simulink model "scenario1_more_complex_new"  (R2020b)
settings: Solver=FixedStepAuto  StartTime=0.0  StopTime=60.0  FixedStep=1e-2  RelTol=1e-3
libraries: simulink x3
settings Model: Creator=Admin  LastModifiedBy=Admin

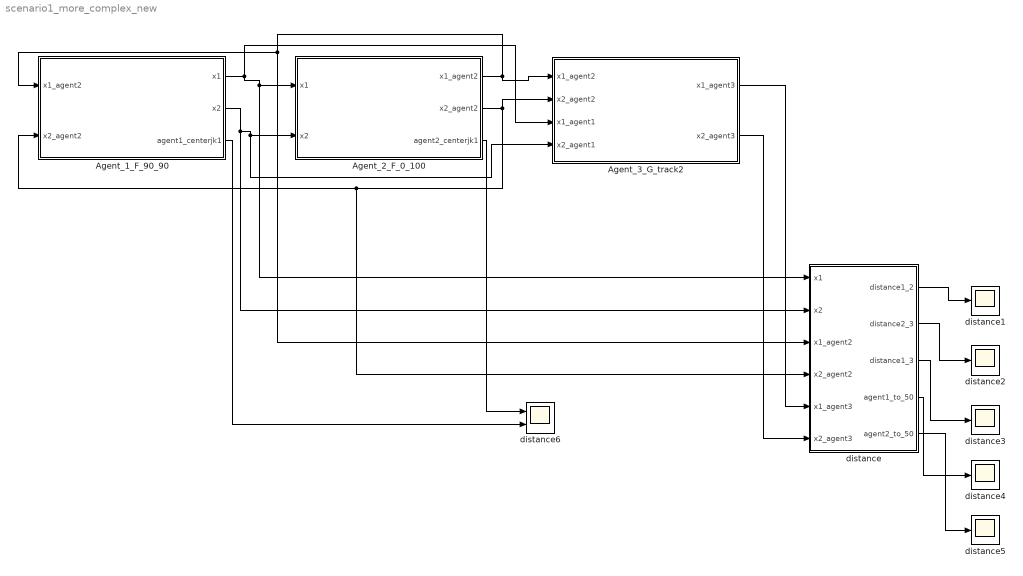
== system scenario1_more_complex_new ==
  Agent_1_F_90_90 : Subsystem
  Agent_2_F_0_100 : Subsystem
  Agent_3_G_track2 : Subsystem
  "distance " : MATLAB Function  TreatAsAtomicUnit=on
  distance{1..5} (5 alike) : Scope
  distance6 : Scope  NumInputPorts=2
  wires:
  Agent_1_F_90_90/1(x1) -> "distance "/1(x1), Agent_2_F_0_100/1(x1), Agent_3_G_track2/3(x1_agent1)
  Agent_1_F_90_90/2(x2) -> "distance "/2(x2), Agent_3_G_track2/4(x2_agent1), Agent_2_F_0_100/2(x2)
  Agent_2_F_0_100/1(x1_agent2) -> Agent_3_G_track2/1(x1_agent2), "distance "/3(x1_agent2), Agent_1_F_90_90/1(x1_agent2)
  Agent_2_F_0_100/2(x2_agent2) -> "distance "/4(x2_agent2), Agent_1_F_90_90/2(x2_agent2), Agent_3_G_track2/2(x2_agent2)
  "distance "/1(distance1_2) -> distance1/1
  Agent_3_G_track2/1(x1_agent3) -> "distance "/5(x1_agent3)
  Agent_3_G_track2/2(x2_agent3) -> "distance "/6(x2_agent3)
  "distance "/2(distance2_3) -> distance2/1
  "distance "/3(distance1_3) -> distance3/1
  "distance "/4(agent1_to_50) -> distance4/1
  "distance "/5(agent2_to_50) -> distance5/1
  Agent_2_F_0_100/3(agent2_centerjk1) -> distance6/1
  Agent_1_F_90_90/3(agent1_centerjk1) -> distance6/2

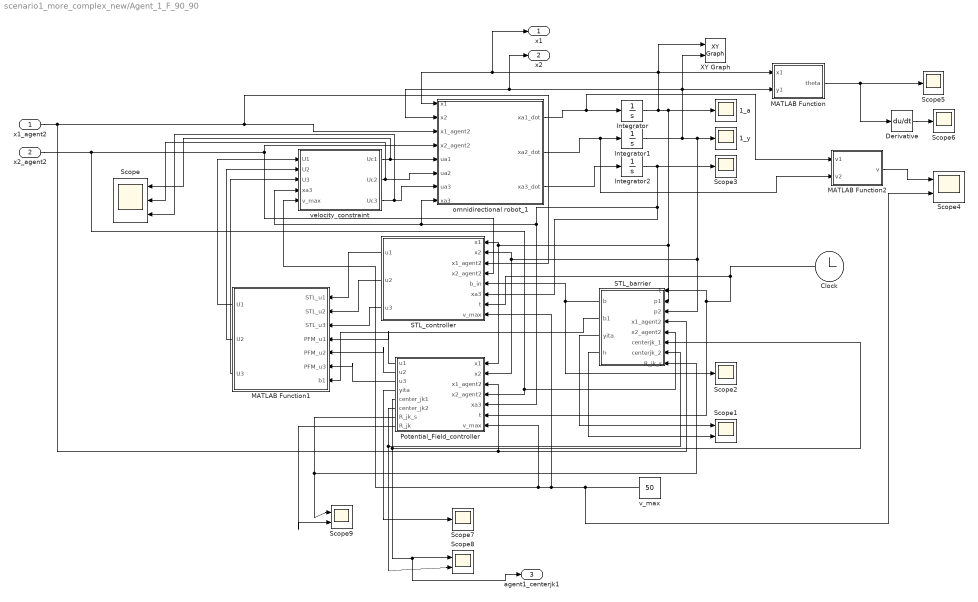
== system scenario1_more_complex_new/Agent_1_F_90_90 ==
  x1_agent2 : Inport
  x2_agent2 : Inport  Port=2
  1_a : Scope
  1_y : Scope
  Clock : Clock
  Derivative : Derivative
  Integrator : Integrator
  Integrator1 : Integrator
  Integrator2 : Integrator
  MATLAB Function : MATLAB Function  TreatAsAtomicUnit=on
  MATLAB Function1 : MATLAB Function  TreatAsAtomicUnit=on
  MATLAB Function2 : MATLAB Function  TreatAsAtomicUnit=on
  Potential_Field_controller : MATLAB Function  TreatAsAtomicUnit=on
  "STL_barrier " : MATLAB Function  TreatAsAtomicUnit=on
  STL_controller : MATLAB Function  TreatAsAtomicUnit=on
  Scope : Scope  NumInputPorts=3
  Scope{1,4,8..9} (4 alike) : Scope  NumInputPorts=2
  Scope{2..3,5..7} (5 alike) : Scope
  XY Graph : simulink/Sinks/XY Graph  xmin=-15  xmax=100  ymin=-15  ymax=100  st=0.01
  omnidirectional robot_1 : MATLAB Function  TreatAsAtomicUnit=on
  v_max : Constant  Value=50
  velocity_constraint : MATLAB Function  TreatAsAtomicUnit=on
  x1 : Outport
  x2 : Outport  Port=2
  agent1_centerjk1 : Outport  Port=3
  wires:
  MATLAB Function/1(theta) -> Derivative/1, Scope5/1
  MATLAB Function1/3(U3) -> velocity_constraint/3(U3)
  "STL_barrier "/1(b) -> Scope2/1, STL_controller/5(b_in)
  Potential_Field_controller/3(u3) -> MATLAB Function1/6(PFM_u3)
  STL_controller/2(u2) -> MATLAB Function1/2(STL_u2)
  Integrator2/1 -> Potential_Field_controller/5(xa3), velocity_constraint/4(xa3), omnidirectional robot_1/8(xa3), STL_controller/6(xa3), Scope3/1
  Integrator1/1 -> x2/1, omnidirectional robot_1/2(x2), MATLAB Function/2(y1), XY Graph/2, "STL_barrier "/3(p2), Potential_Field_controller/2(x2), STL_controller/2(x2), 1_y/1
  Potential_Field_controller/1(u1) -> MATLAB Function1/4(PFM_u1)
  "STL_barrier "/3(yita) -> Scope1/1
  "STL_barrier "/4(h) -> Scope1/2
  omnidirectional robot_1/1(xa1_dot) -> MATLAB Function2/1(v1), Integrator/1
  STL_controller/1(u1) -> MATLAB Function1/1(STL_u1)
  "STL_barrier "/2(b1) -> MATLAB Function1/7(b1)
  STL_controller/3(u3) -> MATLAB Function1/3(STL_u3)
  omnidirectional robot_1/3(xa3_dot) -> Integrator2/1
  Clock/1 -> Potential_Field_controller/6(t), "STL_barrier "/1(t), STL_controller/7(t)
  MATLAB Function1/1(U1) -> velocity_constraint/1(U1)
  Derivative/1 -> Scope6/1
  omnidirectional robot_1/2(xa2_dot) -> MATLAB Function2/2(v2), Integrator1/1
  Potential_Field_controller/2(u2) -> MATLAB Function1/5(PFM_u2)
  MATLAB Function1/2(U2) -> velocity_constraint/2(U2)
  Integrator/1 -> x1/1, omnidirectional robot_1/1(x1), MATLAB Function/1(x1), XY Graph/1, "STL_barrier "/2(p1), Potential_Field_controller/1(x1), STL_controller/1(x1), 1_a/1
  x1_agent2/1 -> "STL_barrier "/4(x1_agent2), Potential_Field_controller/3(x1_agent2), STL_controller/3(x1_agent2), omnidirectional robot_1/3(x1_agent2)
  x2_agent2/1 -> Potential_Field_controller/4(x2_agent2), "STL_barrier "/5(x2_agent2), omnidirectional robot_1/4(x2_agent2), STL_controller/4(x2_agent2)
  MATLAB Function2/1(v) -> Scope4/1
  velocity_constraint/1(Uc1) -> Scope/1, omnidirectional robot_1/5(ua1)
  velocity_constraint/2(Uc2) -> omnidirectional robot_1/6(ua2), Scope/2
  velocity_constraint/3(Uc3) -> Scope/3, omnidirectional robot_1/7(ua3)
  v_max/1 -> Scope4/2, STL_controller/8(v_max), velocity_constraint/5(v_max), Potential_Field_controller/7(v_max)
  Potential_Field_controller/4(yita) -> Scope7/1
  Potential_Field_controller/6(center_jk2) -> "STL_barrier "/7(centerjk_2), Scope8/2
  Potential_Field_controller/7(R_jk_s) -> "STL_barrier "/8(R_jk_s), Scope9/1
  Potential_Field_controller/8(R_jk) -> Scope9/2
  Potential_Field_controller/5(center_jk1) -> agent1_centerjk1/1, Scope8/1, "STL_barrier "/6(centerjk_1)

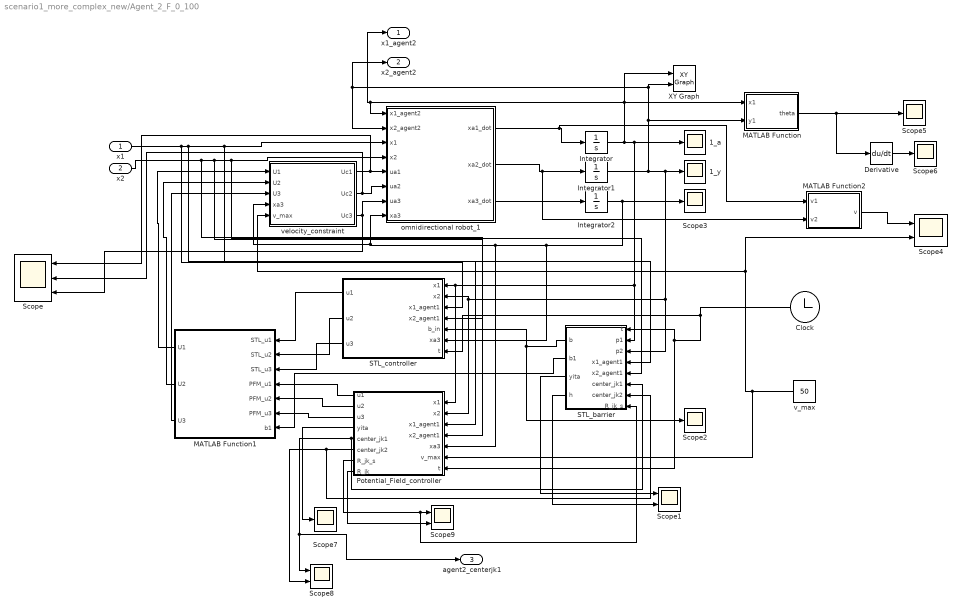
== system scenario1_more_complex_new/Agent_2_F_0_100 ==
  x1 : Inport
  x2 : Inport  Port=2
  1_a : Scope
  1_y : Scope
  Clock : Clock
  Derivative : Derivative
  Integrator : Integrator  InitialCondition=100
  Integrator1 : Integrator
  Integrator2 : Integrator
  MATLAB Function : MATLAB Function  TreatAsAtomicUnit=on
  MATLAB Function1 : MATLAB Function  TreatAsAtomicUnit=on
  MATLAB Function2 : MATLAB Function  TreatAsAtomicUnit=on
  Potential_Field_controller : MATLAB Function  TreatAsAtomicUnit=on
  "STL_barrier " : MATLAB Function  TreatAsAtomicUnit=on
  STL_controller : MATLAB Function  TreatAsAtomicUnit=on
  Scope : Scope  NumInputPorts=3
  Scope{1,4,8..9} (4 alike) : Scope  NumInputPorts=2
  Scope{2..3,5..7} (5 alike) : Scope
  XY Graph : simulink/Sinks/XY Graph  xmin=-15  xmax=100  ymin=-15  ymax=100  st=0.01
  omnidirectional robot_1 : MATLAB Function  TreatAsAtomicUnit=on
  v_max : Constant  Value=50
  velocity_constraint : MATLAB Function  TreatAsAtomicUnit=on
  x1_agent2 : Outport
  x2_agent2 : Outport  Port=2
  agent2_centerjk1 : Outport  Port=3
  wires:
  MATLAB Function/1(theta) -> Derivative/1, Scope5/1
  MATLAB Function1/3(U3) -> velocity_constraint/3(U3)
  "STL_barrier "/1(b) -> Scope2/1, STL_controller/5(b_in)
  Potential_Field_controller/3(u3) -> MATLAB Function1/6(PFM_u3)
  STL_controller/2(u2) -> MATLAB Function1/2(STL_u2)
  Integrator2/1 -> Potential_Field_controller/5(xa3), velocity_constraint/4(xa3), omnidirectional robot_1/8(xa3), STL_controller/6(xa3), Scope3/1
  Integrator1/1 -> x2_agent2/1, omnidirectional robot_1/2(x2_agent2), XY Graph/2, MATLAB Function/2(y1), "STL_barrier "/3(p2), Potential_Field_controller/2(x2), STL_controller/2(x2), 1_y/1
  Potential_Field_controller/1(u1) -> MATLAB Function1/4(PFM_u1)
  Integrator/1 -> x1_agent2/1, omnidirectional robot_1/1(x1_agent2), MATLAB Function/1(x1), XY Graph/1, "STL_barrier "/2(p1), Potential_Field_controller/1(x1), STL_controller/1(x1), 1_a/1
  "STL_barrier "/3(yita) -> Scope1/1
  "STL_barrier "/4(h) -> Scope1/2
  omnidirectional robot_1/1(xa1_dot) -> MATLAB Function2/1(v1), Integrator/1
  STL_controller/1(u1) -> MATLAB Function1/1(STL_u1)
  "STL_barrier "/2(b1) -> MATLAB Function1/7(b1)
  STL_controller/3(u3) -> MATLAB Function1/3(STL_u3)
  omnidirectional robot_1/3(xa3_dot) -> Integrator2/1
  Clock/1 -> Potential_Field_controller/7(t), "STL_barrier "/1(t), STL_controller/7(t)
  MATLAB Function1/1(U1) -> velocity_constraint/1(U1)
  Derivative/1 -> Scope6/1
  omnidirectional robot_1/2(xa2_dot) -> MATLAB Function2/2(v2), Integrator1/1
  Potential_Field_controller/2(u2) -> MATLAB Function1/5(PFM_u2)
  MATLAB Function1/2(U2) -> velocity_constraint/2(U2)
  x1/1 -> STL_controller/3(x1_agent1), Potential_Field_controller/3(x1_agent1), "STL_barrier "/4(x1_agent1), omnidirectional robot_1/3(x1)
  x2/1 -> STL_controller/4(x2_agent1), Potential_Field_controller/4(x2_agent1), "STL_barrier "/5(x2_agent1), omnidirectional robot_1/4(x2)
  MATLAB Function2/1(v) -> Scope4/1
  v_max/1 -> Potential_Field_controller/6(v_max), Scope4/2, velocity_constraint/5(v_max)
  velocity_constraint/1(Uc1) -> Scope/1, omnidirectional robot_1/5(ua1)
  velocity_constraint/2(Uc2) -> Scope/2, omnidirectional robot_1/6(ua2)
  velocity_constraint/3(Uc3) -> Scope/3, omnidirectional robot_1/7(ua3)
  Potential_Field_controller/4(yita) -> Scope7/1
  Potential_Field_controller/5(center_jk1) -> "STL_barrier "/6(center_jk1), Scope8/1, agent2_centerjk1/1
  Potential_Field_controller/6(center_jk2) -> "STL_barrier "/7(center_jk2), Scope8/2
  Potential_Field_controller/7(R_jk_s) -> "STL_barrier "/8(R_jk_s), Scope9/1
  Potential_Field_controller/8(R_jk) -> Scope9/2

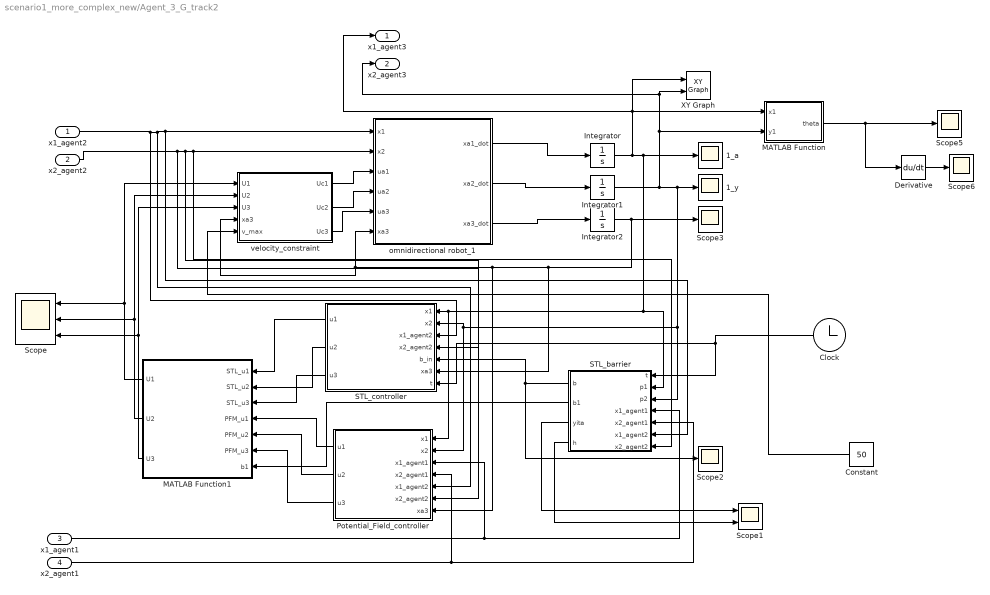
== system scenario1_more_complex_new/Agent_3_G_track2 ==
  x1_agent2 : Inport
  x2_agent2 : Inport  Port=2
  x1_agent1 : Inport  Port=3
  x2_agent1 : Inport  Port=4
  1_a : Scope
  1_y : Scope
  Clock : Clock
  Constant : Constant  Value=50
  Derivative : Derivative
  Integrator : Integrator  InitialCondition=100
  Integrator1 : Integrator  InitialCondition=50
  Integrator2 : Integrator
  MATLAB Function : MATLAB Function  TreatAsAtomicUnit=on
  MATLAB Function1 : MATLAB Function  TreatAsAtomicUnit=on
  Potential_Field_controller : MATLAB Function  TreatAsAtomicUnit=on
  "STL_barrier " : MATLAB Function  TreatAsAtomicUnit=on
  STL_controller : MATLAB Function  TreatAsAtomicUnit=on
  Scope : Scope  NumInputPorts=3
  Scope1 : Scope  NumInputPorts=2
  Scope{2..3,5..6} (4 alike) : Scope
  XY Graph : simulink/Sinks/XY Graph  xmin=-15  xmax=100  ymin=-15  ymax=100  st=0.01
  omnidirectional robot_1 : MATLAB Function  TreatAsAtomicUnit=on
  velocity_constraint : MATLAB Function  TreatAsAtomicUnit=on
  x1_agent3 : Outport
  x2_agent3 : Outport  Port=2
  wires:
  MATLAB Function/1(theta) -> Derivative/1, Scope5/1
  MATLAB Function1/3(U3) -> velocity_constraint/3(U3), Scope/3
  "STL_barrier "/1(b) -> STL_controller/5(b_in), Scope2/1
  Potential_Field_controller/3(u3) -> MATLAB Function1/6(PFM_u3)
  STL_controller/2(u2) -> MATLAB Function1/2(STL_u2)
  Integrator2/1 -> Potential_Field_controller/7(xa3), omnidirectional robot_1/6(xa3), velocity_constraint/4(xa3), STL_controller/6(xa3), Scope3/1
  Integrator1/1 -> x2_agent3/1, XY Graph/2, MATLAB Function/2(y1), "STL_barrier "/3(p2), Potential_Field_controller/2(x2), STL_controller/2(x2), 1_y/1
  Potential_Field_controller/1(u1) -> MATLAB Function1/4(PFM_u1)
  Integrator/1 -> x1_agent3/1, MATLAB Function/1(x1), XY Graph/1, "STL_barrier "/2(p1), Potential_Field_controller/1(x1), STL_controller/1(x1), 1_a/1
  "STL_barrier "/3(yita) -> Scope1/1
  "STL_barrier "/4(h) -> Scope1/2
  omnidirectional robot_1/1(xa1_dot) -> Integrator/1
  STL_controller/1(u1) -> MATLAB Function1/1(STL_u1)
  "STL_barrier "/2(b1) -> MATLAB Function1/7(b1)
  STL_controller/3(u3) -> MATLAB Function1/3(STL_u3)
  omnidirectional robot_1/3(xa3_dot) -> Integrator2/1
  Clock/1 -> "STL_barrier "/1(t), STL_controller/7(t)
  MATLAB Function1/1(U1) -> velocity_constraint/1(U1), Scope/1
  Derivative/1 -> Scope6/1
  omnidirectional robot_1/2(xa2_dot) -> Integrator1/1
  Potential_Field_controller/2(u2) -> MATLAB Function1/5(PFM_u2)
  MATLAB Function1/2(U2) -> velocity_constraint/2(U2), Scope/2
  x1_agent2/1 -> STL_controller/3(x1_agent2), Potential_Field_controller/5(x1_agent2), "STL_barrier "/6(x1_agent2), omnidirectional robot_1/1(x1)
  x2_agent2/1 -> STL_controller/4(x2_agent2), Potential_Field_controller/6(x2_agent2), "STL_barrier "/7(x2_agent2), omnidirectional robot_1/2(x2)
  x1_agent1/1 -> Potential_Field_controller/3(x1_agent1), "STL_barrier "/4(x1_agent1)
  x2_agent1/1 -> Potential_Field_controller/4(x2_agent1), "STL_barrier "/5(x2_agent1)
  Constant/1 -> velocity_constraint/5(v_max)
  velocity_constraint/1(Uc1) -> omnidirectional robot_1/3(ua1)
  velocity_constraint/2(Uc2) -> omnidirectional robot_1/4(ua2)
  velocity_constraint/3(Uc3) -> omnidirectional robot_1/5(ua3)

== matlab function scenario1_more_complex_new/Agent_2_F_0_100/MATLAB Function ==
  data: x1 input; theta output; y1 input
function theta = fcn(x1, y1)
theta=atan2(y1,x1);

== matlab function scenario1_more_complex_new/Agent_2_F_0_100/MATLAB Function1 ==
  data: STL_u1 input; U1 output; STL_u2 input; STL_u3 input; PFM_u1 input; PFM_u2 input; PFM_u3 input; b1 input; U2 output; U3 output
function [U1,U2,U3] = fcn(STL_u1,STL_u2,STL_u3,PFM_u1,PFM_u2,PFM_u3,b1)
U_goal=[STL_u1;STL_u2;STL_u3];
U_obs=[PFM_u1;PFM_u2;PFM_u3];
k=0.15;
lambda=1-exp(-k*max(b1,0));
U=lambda*U_goal+(1-lambda)*U_obs;
U1=0;U2=0;U3=0;
U1=U(1,1);
U2=U(2,1);
U3=U(3,1);

== matlab function scenario1_more_complex_new/distance  ==
  data: x1 input; distance1_2 output; x2 input; x1_agent2 input; x2_agent2 input; x1_agent3 input; x2_agent3 input; distance2_3 output; distance1_3 output; agent1_to_50 output; agent2_to_50 output
function [distance1_2,distance2_3,distance1_3,agent1_to_50,agent2_to_50] = fcn(x1,x2,x1_agent2,x2_agent2,x1_agent3,x2_agent3)
distance1_2=sqrt((x1-x1_agent2)^2+(x2-x2_agent2)^2);
distance2_3=sqrt((x1_agent2-x1_agent3)^2+(x2_agent2-x2_agent3)^2);
distance1_3=sqrt((x1-x1_agent3)^2+(x2-x2_agent3)^2);
agent1_to_50=sqrt((x1-50)^2+(x2-50)^2);
agent2_to_50=sqrt((x1_agent2-50)^2+(x2_agent2-50)^2);

== matlab function scenario1_more_complex_new/Agent_2_F_0_100/STL_barrier  ==
  data: b output; b1 output; yita output; h output; t input; p1 input; p2 input; x1_agent1 input; x2_agent1 input; center_jk1 input; center_jk2 input; R_jk_s input
function [b,b1,yita,h] = fcn(t,p1,p2,x1_agent1, x2_agent1, center_jk1,center_jk2,R_jk_s)
if t<20
    d1=0;
    d2=100;
elseif t>=20 && t<40
    d1=90;
    d2=90;
else
    d1=0;
    d2=0;
end
    

obs1=50;
obs2=50;

if t<20
    b=145*exp(-0.24*t)+5-sqrt( (p1-d1)^2 + (p2-d2)^2 );
    yita=-145*exp(-0.24*t)+5;
    h=10-sqrt( (p1-d1)^2 + (p2-d2)^2 );
elseif t>=20 && t<40
   b=90*exp(-0.208*(t-20))+5-sqrt( (p1-d1)^2 + (p2-d2)^2 );
   yita=-90*exp(-0.208*(t-20))+5;
   h=10-sqrt( (p1-d1)^2 + (p2-d2)^2 );
else
   b=135*exp(-0.235*(t-40))+5-sqrt( (p1-d1)^2 + (p2-d2)^2 );
   yita=-135*exp(-0.235*(t-40))+5;
   h=10-sqrt( (p1-d1)^2 + (p2-d2)^2 );    
end
b11=sqrt( (p1-obs1)^2 + (p2-obs2)^2 )-20;%collision avoidence with (50,50)
b12=sqrt( (p1-x1_agent1)^2 + (p2-x2_agent1)^2 )-6;%collision avoidence with agent1
b13=sqrt( (p1-center_jk1)^2 + (p2-center_jk2)^2 )-R_jk_s;%collision avoidence with agent1
b14=sqrt( (p1-60)^2 + (p2-80)^2 )-15;
b15=sqrt( (p1-10)^2 + (p2-70)^2 )-10;
if R_jk_s==0
b1=-(1/20)*log(exp(-20*b11)+exp(-20*b12)+exp(-20*b14)+exp(-20*b15));%+log(2);
else
b1=-(1/20)*log(exp(-20*b11)+exp(-20*b12)+exp(-20*b13)+exp(-20*b14)+exp(-20*b15));%+log(2);
end

== matlab function scenario1_more_complex_new/Agent_2_F_0_100/STL_controller ==
  data: x1 input; x2 input; x1_agent1 input; x2_agent1 input; b_in input; u1 output; xa3 input; u2 output; u3 output; t input
function [u1,u2,u3]= fcn(x1, x2,x1_agent1,x2_agent1, b_in, xa3,t)
%Note：x are the position of agent2(myself), and x_agent1 is from another agent
coder.extrinsic('quadoptimizer');
%coder.extrinsic('save');
if t<20
d1=0; d2=100;
elseif t>=20 && t<40
d1=90; d2=90;
else
d1=0; d2=0;
end
partial_b=(1/2)*((x1-d1)^2+(x2-d2)^2)^(-1/2);
partial_b_x=[-2*partial_b*(x1-d1),-2*partial_b*(x2-d2),0];


Li=0.2;
Bi=[0,cos(pi/6),-cos(pi/6);
    -1,sin(pi/6),sin(pi/6);
    Li,Li,Li;];

R1=[cos(xa3),-sin(xa3),0;
    sin(xa3),cos(xa3),0;
    0,0,1;];
R=0.02;
gx=R1*inv(Bi')*R;

A=partial_b_x*gx;
% A=[A;-gx];

H=[1,0,0;0,1,0;0,0,1];
%H=[1];
if t<20
   b=2*b_in-0.24*125*exp(-0.24*t)-4;
elseif t>=20 && t<40
   b=2*b_in-0.208*90*exp(-0.208*(t-20))-4;
else
   b=2*b_in-0.235*135*exp(-0.235*(t-40))-4; 
end
% b=[b;5000;5000;5000];


u1=0;u2=0;u3=0;
U=quadoptimizer(H,b,A);

%U=quadprod(H,[],-A,b);

u1=U(1,1);
u2=U(2,1);
u3=U(3,1);

== matlab function scenario1_more_complex_new/Agent_2_F_0_100/omnidirectional robot_1 ==
  data: x1_agent2 input; x2_agent2 input; x1 input; x2 input; ua1 input; xa1_dot output; ua2 input; ua3 input; xa3 input; xa2_dot output; xa3_dot output
function [xa1_dot,xa2_dot,xa3_dot]= fcn(x1_agent2,x2_agent2,x1,x2,ua1,ua2,ua3,xa3)

Li=0.2;
Bi=[0,cos(pi/6),-cos(pi/6);
    -1,sin(pi/6),sin(pi/6);
    Li,Li,Li;];

R1=[cos(xa3),-sin(xa3),0;
    sin(xa3),cos(xa3),0;
    0,0,1;];
R=0.02;
A=R1*inv(Bi')*R*[ua1;ua2;ua3];
xa1_dot=A(1,1);
xa2_dot=A(2,1);
xa3_dot=A(3,1);

== matlab function scenario1_more_complex_new/Agent_2_F_0_100/Potential_Field_controller ==
  data: x1 input; x2 input; x1_agent1 input; x2_agent1 input; u1 output; xa3 input; u2 output; u3 output; v_max input; yita output; center_jk1 output; center_jk2 output; R_jk_s output; R_jk output; t input
function [u1,u2,u3,yita,center_jk1,center_jk2,R_jk_s,R_jk] = fcn(x1, x2, x1_agent1,x2_agent1, xa3,v_max,t)
coder.extrinsic('Calculate_gradient');
coder.extrinsic('Calculate_gradient_V2');
coder.extrinsic('Calculate_gradient_V1_yita');
coder.extrinsic('Calculate_gradient_static_d_1');
coder.extrinsic('Calculate_gradient_static_d_2');
coder.extrinsic('compute_convex_hull');
coder.extrinsic('PVF_optimizer');
coder.extrinsic('add_random');
yita=0;
center_jk1=0;center_jk2=0;
A1=[-1,0;0,-1];
if t<20
    F=[0,200];
elseif t>=20 && t<40
    F=[180,180];
else 
   F=[0,0]; 
end
obs=[50,50];
Robs_s=20;R1_s=6;
r_obs=16;d1=3;
R_jk_s=0;R_jk=0
distance=sqrt((x1-0)^2+(x2-100)^2);
gradient_x=0;gradient_y=0;
Dgradient_x=0;Dgradient_y=0;D1gradient_x=0;D1gradient_y=0;D2gradient_x=0;D2gradient_y=0;
[gradient_x,gradient_y]=Calculate_gradient(x1,x2,A1,F,50,50,Robs_s);
[Dgradient_x,Dgradient_y]=Calculate_gradient_V2(x1,x2,A1,F,x1_agent1,x2_agent1,R1_s);
[D1gradient_x,D1gradient_y]=Calculate_gradient_static_d_1(x1,x2,A1,F,60,85,15);
[D2gradient_x,D2gradient_y]=Calculate_gradient_static_d_2(x1,x2,A1,F,10,70,10);
agent_distance=sqrt((x1-x1_agent1)^2+(x2-x2_agent1)^2);%the distance between 1 and 2.
if t>20
gradient_x=gradient_x+D1gradient_x;
gradient_y=gradient_y+D1gradient_y;
else
gradient_x=gradient_x+D2gradient_x;
gradient_y=gradient_y+D2gradient_y;
end
% gradient_x=Gradient(1,1);
% gradient_y=Gradient(1,2);
gradient_z=0;

if agent_distance>50
     Gradient_all=[gradient_x;gradient_y;gradient_z];
else 
     gradient_x=gradient_x+Dgradient_x;
     gradient_y=gradient_y+Dgradient_y;
     Gradient_all=[gradient_x;gradient_y;gradient_z];
end
% if agent_distance>40
%     Gradient_all=[gradient_x;gradient_y;gradient_z];
% else %collision avoidence with agent 2
%      if sqrt((x1_agent1-obs(1,1))^2+(x2_agent1-obs(1,2))^2)>Robs_s+R1_s %compute if intersection happens,No intersecdtion
%          gradient_x=gradient_x+Dgradient_x;
%          gradient_y=gradient_y+Dgradient_y;
%          Gradient_all=[gradient_x;gradient_y;gradient_z];
%      else %intersecdtion happens
%          center_jk1=0; center_jk2=0; R_jk=0;flg_jk=0;
%          [center_jk1, center_jk2, R_jk,flg_jk]=compute_convex_hull(x1,x2,obs(1,1), obs(1,2), x1_agent1, x2_agent1,r_obs,d1);
%           if sqrt((x1-center_jk1)^2+(x2-center_jk2)^2)<R_jk %inside the convexhull
%                [Dgradient_x,Dgradient_y]=Calculate_gradient_V1(x1,x2,A1,F,x1_agent2,x2_agent2,R2_s*exp(-2*v_max*(t-t0)));
%                   gradient_x=gradient_x;%+Dgradient_x;
%                   gradient_y=gradient_y;%+Dgradient_y;
%                   Gradient_all=[gradient_x;gradient_y;gradient_z];
%                   center_jk1=10; center_jk2=0;
%           else %outside the convexhull
%               if flg_jk==1 %outside and nomial need to be built
%                R_jk_s=(R_jk/d1)*R1_s;  
%                    R_jk_s=sqrt((x1-center_jk1)^2+(x2-center_jk2)^2);
%                    R_jk_s=50;
%                    yita= ( (v_max+50*0.6+2)*R_jk^3 )/( 50*(1- (R_jk/R_jk_s) ) );
%                    Djkgradient_x=0;Djkgradient_y=0;
%                    [Djkgradient_x,Djkgradient_y]=Calculate_gradient_V1_yita(x1,x2,A1,F,center_jk1,center_jk2,R_jk_s,yita);
%                     gradient_x=gradient_x+Dgradient_x+Djkgradient_x;
%                     gradient_y=gradient_y+Dgradient_y+Djkgradient_y;
%                     Gradient_all=[gradient_x;gradient_y;gradient_z];
%               else %%outside and nomialdo not need to be built
%                     gradient_x=gradient_x+Dgradient_x;
%                     gradient_y=gradient_y+Dgradient_y;
%                     Gradient_all=[gradient_x;gradient_y;gradient_z];
%               end
%           end
%      end
% end
             

Li=0.2;
Bi=[0,cos(pi/6),-cos(pi/6);
    -1,sin(pi/6),sin(pi/6);
    Li,Li,Li;];

R1=[cos(xa3),-sin(xa3),0;
    sin(xa3),cos(xa3),0;
    0,0,1;];
R=0.02;

gx=R1*inv(Bi')*R;
A=Gradient_all'*gx;
% A=[A;-gx];

%H=[1];
%H=[1,0;0,1];
%H=[0,0,0;0,0,0;0,0,0];
% H=[1,0,0;0,1,0;0,0,1];
 H=(1/2)*gx'*gx;
b=[0];
% b=[0;5000;5000;5000];
Gain=50;
Gradient_final=Gain*Gradient_all;
F=[-2*gx'*Gradient_final];
%=[];
u1=0;u2=0;u3=0;
U=PVF_optimizer(H,b,A,F,distance,gradient_x,gradient_y);

u1=U(1,1);
u2=U(2,1);
u3=U(3,1);

== matlab function scenario1_more_complex_new/Agent_1_F_90_90/STL_barrier  ==
  data: b output; b1 output; yita output; h output; t input; p1 input; p2 input; x1_agent2 input; x2_agent2 input; centerjk_1 input; centerjk_2 input; R_jk_s input
function [b,b1,yita,h] = fcn(t,p1,p2, x1_agent2, x2_agent2,centerjk_1,centerjk_2,R_jk_s)
if t<20
    d1=90;
    d2=90;
elseif t>=20 && t<40
    d1=0;
    d2=100;
else
    d1=100;
    d2=0;  
end

obs1=50;
obs2=50;
if t<20
b=125*exp(-0.2295*t)+5-sqrt( (p1-d1)^2 + (p2-d2)^2 );
yita=-125*exp(-0.2295*t)+5;
h=10-sqrt( (p1-d1)^2 + (p2-d2)^2 );
elseif t>=20 && t<40
    b=90*exp(-0.208*(t-20))+5-sqrt( (p1-d1)^2 + (p2-d2)^2 );
   yita=-90*exp(-0.2295*(t-20))+5;
    h=10-sqrt( (p1-d1)^2 + (p2-d2)^2 );
else
   b=145*exp(-0.24*(t-40))+5-sqrt( (p1-d1)^2 + (p2-d2)^2 );
   yita=-145*exp(-0.24*(t-40))+5;
   h=10-sqrt( (p1-d1)^2 + (p2-d2)^2 );
end
b11=sqrt( (p1-x1_agent2)^2 + (p2-x2_agent2)^2 )-10 %collision avoidence with agent2
b12=sqrt( (p1-obs1)^2 + (p2-obs2)^2 )-20;%collision avoidence with obstacle (50,50)
b13=sqrt( (p1-centerjk_1)^2 + (p2-centerjk_2)^2 )-R_jk_s;%collision avoidence with nominal
b14=sqrt( (p1-60)^2 + (p2-80)^2 )-15; %static dynamic obstacle
b15=sqrt( (p1-10)^2 + (p2-70)^2 )-10; %static dynamic obstacle
if R_jk_s==0

b1=-(1/20)*log(exp(-20*b11)+exp(-20*b12)+exp(-20*b14)+exp(-20*b15));%+log(2);

else
 b1=-(1/20)*log(exp(-20*b11)+exp(-20*b12)+exp(-20*b13)+exp(-20*b14)+exp(-20*b15));%+log(2);   
end

== matlab function scenario1_more_complex_new/Agent_3_G_track2/MATLAB Function ==
  data: x1 input; theta output; y1 input
function theta = fcn(x1, y1)
theta=atan2(y1,x1);

== matlab function scenario1_more_complex_new/Agent_3_G_track2/MATLAB Function1 ==
  data: STL_u1 input; U1 output; STL_u2 input; STL_u3 input; PFM_u1 input; PFM_u2 input; PFM_u3 input; b1 input; U2 output; U3 output
function [U1,U2,U3] = fcn(STL_u1,STL_u2,STL_u3,PFM_u1,PFM_u2,PFM_u3,b1)
U_goal=[STL_u1;STL_u2;STL_u3];
U_obs=[PFM_u1;PFM_u2;PFM_u3];
k=0.3;
lambda=1-exp(-k*max(b1,0));
U=lambda*U_goal+(1-lambda)*U_obs;
%  U=U_obs;
U1=0;U2=0;U3=0;
U1=U(1,1);
U2=U(2,1);
U3=U(3,1);

== matlab function scenario1_more_complex_new/Agent_3_G_track2/Potential_Field_controller ==
  data: x1 input; x2 input; x1_agent1 input; x2_agent1 input; x1_agent2 input; x2_agent2 input; u1 output; xa3 input; u2 output; u3 output
function [u1,u2,u3] = fcn(x1, x2,x1_agent1,x2_agent1, x1_agent2,x2_agent2, xa3)
coder.extrinsic('Calculate_gradient');
coder.extrinsic('PVF_optimizer');
coder.extrinsic('Calculate_gradient_V1');
coder.extrinsic('Calculate_gradient_static_d_2');
coder.extrinsic('add_random');
A1=[-1,0;0,-1];
F=[2*x1_agent2,2*x2_agent2];
distance=sqrt((x1-0)^2+(x2-100)^2);%distance to (0,100).not useful in this case
distance_1_3=sqrt((x1_agent1-x1)^2+(x2_agent1-x2)^2);
gradient_x=0;gradient_y=0;
Dgradient_x=0;Dgradient_y=0;
D2gradient_x=0;D2gradient_y=0;
[gradient_x,gradient_y]=Calculate_gradient(x1,x2,A1,F,50,50,20);
[Dgradient_x,Dgradient_y]=Calculate_gradient_V1(x1,x2,A1,F,x1_agent1,x2_agent1,10);
[D2gradient_x,D2gradient_y]=Calculate_gradient_static_d_2(x1,x2,A1,F,10,70,10);
gradient_z=0;
if distance_1_3 > 5
    Gradient_all=[gradient_x+D2gradient_x;gradient_y+D2gradient_y;gradient_z];
else %collision avoidence with agent 1
  gradient_x=  gradient_x+Dgradient_x;
  gradient_y= gradient_y+Dgradient_y;
  Gradient_all=[gradient_x+D2gradient_x;gradient_y+D2gradient_y;gradient_z];
end

Li=0.2;
Bi=[0,cos(pi/6),-cos(pi/6);
    -1,sin(pi/6),sin(pi/6);
    Li,Li,Li;];

R1=[cos(xa3),-sin(xa3),0;
    sin(xa3),cos(xa3),0;
    0,0,1;];
R=0.02;
Distance=sqrt((x1-x1_agent2)^2+(x2-x2_agent2)^2);
gx=R1*inv(Bi')*R;
A=Gradient_all'*gx;

%H=[1];
%H=[1,0;0,1];
%H=[0,0,0;0,0,0;0,0,0];
% H=[1,0,0;0,1,0;0,0,1];
 H=(1/2)*gx'*gx;
b=[0];
F=[-2*gx'*100*Distance*Gradient_all];
%=[];
u1=0;u2=0;u3=0;
U=PVF_optimizer(H,b,A,F,distance,gradient_x,gradient_y);

u1=U(1,1);
u2=U(2,1);
u3=U(3,1);

== matlab function scenario1_more_complex_new/Agent_3_G_track2/STL_barrier  ==
  data: b output; b1 output; yita output; h output; t input; p1 input; p2 input; x1_agent1 input; x2_agent1 input; x1_agent2 input; x2_agent2 input
function [b,b1,yita,h] = fcn(t,p1,p2,x1_agent1,x2_agent1,x1_agent2,x2_agent2)
d1=0;
d2=100;

obs1=50;
obs2=50;

b=55*exp(-0.525*t)+5-sqrt( (p1-x1_agent2)^2 + (p2-x2_agent2)^2 ); %track agent2
yita=-55*exp(-0.525*t)+5;
h=10-sqrt( (p1-x1_agent2)^2 + (p2-x2_agent2)^2 );
b11=sqrt( (p1-obs1)^2 + (p2-obs2)^2 )-16;%collision avoidence with (50,50)
b12=sqrt( (p1-x1_agent1)^2 + (p2-x2_agent1)^2 )-5;% collision avoidence with agent1 
b1=-(1/20)*log(exp(-20*b11)+exp(-20*b12));

== matlab function scenario1_more_complex_new/Agent_3_G_track2/STL_controller ==
  data: x1 input; x2 input; x1_agent2 input; x2_agent2 input; b_in input; u1 output; xa3 input; u2 output; u3 output; t input
function [u1,u2,u3]= fcn(x1, x2,x1_agent2,x2_agent2, b_in, xa3,t)
%Note：x are the position of agent2(myself), and x_agent1 is from another agent
coder.extrinsic('quadoptimizer');
%coder.extrinsic('save');
d1=0; d2=100;

partial_b=(1/2)*((x1-x1_agent2)^2+(x2-x2_agent2)^2)^(-1/2);
partial_b_x=[-2*partial_b*(x1-x1_agent2),-2*partial_b*(x2-x2_agent2),0];
partial_b_x2=[-2*partial_b*(x1-x1_agent2),-2*partial_b*(x2-x2_agent2)];
pho1=sqrt(partial_b_x2(1,1)^2+partial_b_x2(1,2)^2);

Li=0.2;
Bi=[0,cos(pi/6),-cos(pi/6);
    -1,sin(pi/6),sin(pi/6);
    Li,Li,Li;];

R1=[cos(xa3),-sin(xa3),0;
    sin(xa3),cos(xa3),0;
    0,0,1;];
R=0.02;
gx=R1*inv(Bi')*R;

A=partial_b_x*gx;

H=[1,0,0;0,1,0;0,0,1];
%H=[1];

b=150*b_in-0.525*55*exp(-0.525*t)-50*pho1-20;



u1=0;u2=0;u3=0;
U=quadoptimizer(H,b,A);

%U=quadprod(H,[],-A,b);

u1=U(1,1);
u2=U(2,1);
u3=U(3,1);

== matlab function scenario1_more_complex_new/Agent_3_G_track2/omnidirectional robot_1 ==
  data: x1 input; x2 input; ua1 input; xa1_dot output; ua2 input; ua3 input; xa3 input; xa2_dot output; xa3_dot output
function [xa1_dot,xa2_dot,xa3_dot]= fcn(x1,x2,ua1,ua2,ua3,xa3)

Li=0.2;
Bi=[0,cos(pi/6),-cos(pi/6);
    -1,sin(pi/6),sin(pi/6);
    Li,Li,Li;];

R1=[cos(xa3),-sin(xa3),0;
    sin(xa3),cos(xa3),0;
    0,0,1;];
R=0.02;
A=R1*inv(Bi')*R*[ua1;ua2;ua3];
xa1_dot=A(1,1);
xa2_dot=A(2,1);
xa3_dot=A(3,1);

== matlab function scenario1_more_complex_new/Agent_1_F_90_90/MATLAB Function2 ==
  data: v1 input; v output; v2 input
function v = fcn(v1, v2)
v=sqrt(v1^2+v2^2);

== matlab function scenario1_more_complex_new/Agent_1_F_90_90/velocity_constraint ==
  data: U1 input; Uc1 output; U2 input; U3 input; Uc2 output; Uc3 output; xa3 input; v_max input
function [Uc1,Uc2,Uc3] = fcn(U1,U2,U3,xa3,v_max)

Li=0.2;
Bi=[0,cos(pi/6),-cos(pi/6);
    -1,sin(pi/6),sin(pi/6);
    Li,Li,Li;];

R1=[cos(xa3),-sin(xa3),0;
    sin(xa3),cos(xa3),0;
    0,0,1;];
R=0.02;
gx=R1*inv(Bi')*R;

U=[U1;U2;U3];
V=[0;0;0];
V=gx*U;
if V(1,1)^2+V(2,1)^2<=v_max^2
     U(1,1)= U(1,1);
     U(2,1)= U(2,1);
else 
    U(1,1)=sqrt(v_max^2/(V(1,1)^2+V(2,1)^2))*U(1,1);
    U(2,1)=sqrt(v_max^2/(V(1,1)^2+V(2,1)^2))*U(2,1);
    U(3,1)=sqrt(v_max^2/(V(1,1)^2+V(2,1)^2))*U(3,1);
end

Uc1=U(1,1);
Uc2=U(2,1);
Uc3=U(3,1);

== matlab function scenario1_more_complex_new/Agent_2_F_0_100/velocity_constraint ==
  data: U1 input; Uc1 output; U2 input; U3 input; Uc2 output; Uc3 output; xa3 input; v_max input
function [Uc1,Uc2,Uc3] = fcn(U1,U2,U3,xa3,v_max)

Li=0.2;
Bi=[0,cos(pi/6),-cos(pi/6);
    -1,sin(pi/6),sin(pi/6);
    Li,Li,Li;];

R1=[cos(xa3),-sin(xa3),0;
    sin(xa3),cos(xa3),0;
    0,0,1;];
R=0.02;
gx=R1*inv(Bi')*R;

U=[U1;U2;U3];
V=[0;0;0];
V=gx*U;
if V(1,1)^2+V(2,1)^2<=v_max^2
     U(1,1)= U(1,1);
     U(2,1)= U(2,1);
else 
    U(1,1)=sqrt(v_max^2/(V(1,1)^2+V(2,1)^2))*U(1,1);
    U(2,1)=sqrt(v_max^2/(V(1,1)^2+V(2,1)^2))*U(2,1);
    U(3,1)=sqrt(v_max^2/(V(1,1)^2+V(2,1)^2))*U(3,1);
end

Uc1=U(1,1);
Uc2=U(2,1);
Uc3=U(3,1);

== matlab function scenario1_more_complex_new/Agent_2_F_0_100/MATLAB Function2 ==
  data: v1 input; v output; v2 input
function v = fcn(v1, v2)
v=sqrt(v1^2+v2^2);

== matlab function scenario1_more_complex_new/Agent_3_G_track2/velocity_constraint ==
  data: U1 input; Uc1 output; U2 input; U3 input; Uc2 output; Uc3 output; xa3 input; v_max input
function [Uc1,Uc2,Uc3] = fcn(U1,U2,U3,xa3,v_max)

Li=0.2;
Bi=[0,cos(pi/6),-cos(pi/6);
    -1,sin(pi/6),sin(pi/6);
    Li,Li,Li;];

R1=[cos(xa3),-sin(xa3),0;
    sin(xa3),cos(xa3),0;
    0,0,1;];
R=0.02;
gx=R1*inv(Bi')*R;

U=[U1;U2;U3];
V=[0;0;0];
V=gx*U;
if V(1,1)^2+V(2,1)^2<=v_max^2
     U(1,1)= U(1,1);
     U(2,1)= U(2,1);
else 
    U(1,1)=sqrt(v_max^2/(V(1,1)^2+V(2,1)^2))*U(1,1);
    U(2,1)=sqrt(v_max^2/(V(1,1)^2+V(2,1)^2))*U(2,1);
    U(3,1)=sqrt(v_max^2/(V(1,1)^2+V(2,1)^2))*U(3,1);
end

Uc1=U(1,1);
Uc2=U(2,1);
Uc3=U(3,1);

== matlab function scenario1_more_complex_new/Agent_1_F_90_90/omnidirectional robot_1 ==
  data: x1 input; x2 input; x1_agent2 input; x2_agent2 input; ua1 input; xa1_dot output; ua2 input; ua3 input; xa3 input; xa2_dot output; xa3_dot output
function [xa1_dot,xa2_dot,xa3_dot]= fcn(x1,x2,x1_agent2,x2_agent2,ua1,ua2,ua3,xa3)

Li=0.2;
Bi=[0,cos(pi/6),-cos(pi/6);
    -1,sin(pi/6),sin(pi/6);
    Li,Li,Li;];

R1=[cos(xa3),-sin(xa3),0;
    sin(xa3),cos(xa3),0;
    0,0,1;];
R=0.02;
A=R1*inv(Bi')*R*[ua1;ua2;ua3];
xa1_dot=A(1,1);
xa2_dot=A(2,1);
xa3_dot=A(3,1);

== matlab function scenario1_more_complex_new/Agent_1_F_90_90/STL_controller ==
  data: x1 input; x2 input; x1_agent2 input; x2_agent2 input; b_in input; u1 output; xa3 input; u2 output; u3 output; t input; v_max input
function [u1,u2,u3]= fcn(x1, x2,x1_agent2,x2_agent2, b_in, xa3,t, v_max)
coder.extrinsic('quadoptimizer');
%coder.extrinsic('save');
if t<20
    d1=90; d2=90;
elseif t>=20 && t<40
   d1=0; d2=100; 
else
   d1=100; d2=0; 
end

partial_b=(1/2)*((x1-d1)^2+(x2-d2)^2)^(-1/2);
partial_b_x=[-2*partial_b*(x1-d1),-2*partial_b*(x2-d2),0];


Li=0.2;
Bi=[0,cos(pi/6),-cos(pi/6);
    -1,sin(pi/6),sin(pi/6);
    Li,Li,Li;];

R1=[cos(xa3),-sin(xa3),0;
    sin(xa3),cos(xa3),0;
    0,0,1;];
R=0.02;
gx=R1*inv(Bi')*R;

A=partial_b_x*gx;
% A=[A;-gx];
H=[1,0,0;0,1,0;0,0,1];
%H=[1];
if t<20
    b=1*b_in-0.2295*125*exp(-0.2295*t)-1;
elseif t>=20 && t<40
    b=20*b_in-0.208*90*exp(-0.208*(t-20))-100;
else
    b=20*b_in-0.24*145*exp(-0.24*(t-40))-100;
end
% b=[b;5000;5000;5000];


u1=0;u2=0;u3=0;
U=[0;0;0];
U=quadoptimizer(H,b,A);

%U=quadprod(H,[],-A,b);
% V=[0;0;0];
% V=gx*U;
% if V(1,1)^2+V(2,1)^2<=v_max^2
%      U(1,1)= U(1,1);
%      U(2,1)= U(2,1);
% else 
%     U(1,1)=sqrt(v_max^2/(V(1,1)^2+V(2,1)^2))*U(1,1);
%     U(2,1)=sqrt(v_max^2/(V(1,1)^2+V(2,1)^2))*U(2,1);
% end


u1=U(1,1);
u2=U(2,1);
u3=U(3,1);

== matlab function scenario1_more_complex_new/Agent_1_F_90_90/MATLAB Function ==
  data: x1 input; theta output; y1 input
function theta = fcn(x1, y1)
theta=atan2(y1,x1);

== matlab function scenario1_more_complex_new/Agent_1_F_90_90/Potential_Field_controller ==
  data: x1 input; x2 input; x1_agent2 input; x2_agent2 input; u1 output; xa3 input; t input; u2 output; u3 output; v_max input; yita output; center_jk1 output; center_jk2 output; R_jk_s output; R_jk output
function [u1,u2,u3,yita,center_jk1,center_jk2,R_jk_s,R_jk] = fcn(x1, x2,x1_agent2,x2_agent2, xa3,t,v_max)
coder.extrinsic('Calculate_gradient');
coder.extrinsic('Calculate_gradient_V1');
coder.extrinsic('Calculate_gradient_V1_yita');
coder.extrinsic('Calculate_gradient_static_d_1');
coder.extrinsic('Calculate_gradient_static_d_2');
coder.extrinsic('compute_convex_hull');
coder.extrinsic('PVF_optimizer');
coder.extrinsic('add_random');
yita=0;
center_jk1=0;center_jk2=0;
A1=[-1,0;0,-1];
if t<20
    F=[180,180];
elseif t>=20 && t<40
     F=[0,200];
else
    F=[200,0];
end
obs=[50,50];
Robs_s=20;R2_s=10;
r_obs=16;d2=6;
R_jk_s=0;R_jk=0;
distance=sqrt((x1-90)^2+(x2-90)^2);
agent_distance=sqrt((x1-x1_agent2)^2+(x2-x2_agent2)^2);%the distance between 1 and 2.
gradient_x=0;gradient_y=0;
Dgradient_x=0;Dgradient_y=0;
D1gradient_x=0;D1gradient_y=0;D2gradient_x=0;D2gradient_y=0;
[gradient_x,gradient_y]=Calculate_gradient(x1,x2,A1,F,50,50,Robs_s);
[Dgradient_x,Dgradient_y]=Calculate_gradient_V1(x1,x2,A1,F,x1_agent2,x2_agent2,R2_s);
[D1gradient_x,D1gradient_y]=Calculate_gradient_static_d_1(x1,x2,A1,F,60,85,15);
[D2gradient_x,D2gradient_y]=Calculate_gradient_static_d_2(x1,x2,A1,F,10,70,10);
if t>20
gradient_x=gradient_x+D1gradient_x+D2gradient_x;
gradient_y=gradient_y+D1gradient_y+D2gradient_y;
else
gradient_x=gradient_x;
gradient_y=gradient_y;
end

% gradient_x=Gradient(1,1);
% gradient_y=Gradient(1,2);
gradient_z=0;
if agent_distance>50
     Gradient_all=[gradient_x;gradient_y;gradient_z];
else 
     gradient_x=gradient_x+Dgradient_x;
     gradient_y=gradient_y+Dgradient_y;
     Gradient_all=[gradient_x;gradient_y;gradient_z];
end


Li=0.2;
Bi=[0,cos(pi/6),-cos(pi/6);
    -1,sin(pi/6),sin(pi/6);
    Li,Li,Li;];

R1=[cos(xa3),-sin(xa3),0;
    sin(xa3),cos(xa3),0;
    0,0,1;];
R=0.02;

gx=R1*inv(Bi')*R;
A=Gradient_all'*gx;
% A=[A;-gx];
%H=[1];
%H=[1,0;0,1];
%H=[0,0,0;0,0,0;0,0,0];
% H=[1,0,0;0,1,0;0,0,1];
 H=(1/2)*gx'*gx;
b=[0];
% b=[0;5000;5000;5000];
Gain=50;
Gradient_final=Gain*Gradient_all;
F=[-2*gx'*Gradient_final];
%=[];
u1=0;u2=0;u3=0;
U=PVF_optimizer(H,b,A,F,distance,gradient_x,gradient_y);

u1=U(1,1);
u2=U(2,1);
u3=U(3,1);

== matlab function scenario1_more_complex_new/Agent_1_F_90_90/MATLAB Function1 ==
  data: STL_u1 input; U1 output; STL_u2 input; STL_u3 input; PFM_u1 input; PFM_u2 input; PFM_u3 input; b1 input; U2 output; U3 output
function [U1,U2,U3] = fcn(STL_u1,STL_u2,STL_u3,PFM_u1,PFM_u2,PFM_u3,b1)
U_goal=[STL_u1;STL_u2;STL_u3];
U_obs=[PFM_u1;PFM_u2;PFM_u3];
k=0.15;
lambda=1-exp(-k*max(b1,0));
U=lambda*U_goal+(1-lambda)*U_obs;
U1=0;U2=0;U3=0;
U1=U(1,1);
U2=U(2,1);
U3=U(3,1);
